simulink model "gm_sampleModel1857_sub"  (R2023a)
settings: Solver=VariableStepAuto  StartTime=0.0  StopTime=10.0  RelTol=1e-3
libraries: simulink x2, hdlsllib x1
settings Model: Creator=user1  LastModifiedBy=user1
settings OptimizationCC: BlockReduction=off  ConditionallyExecuteInputs=off
settings DebuggingCC: InheritedTsInSrcMsg=none

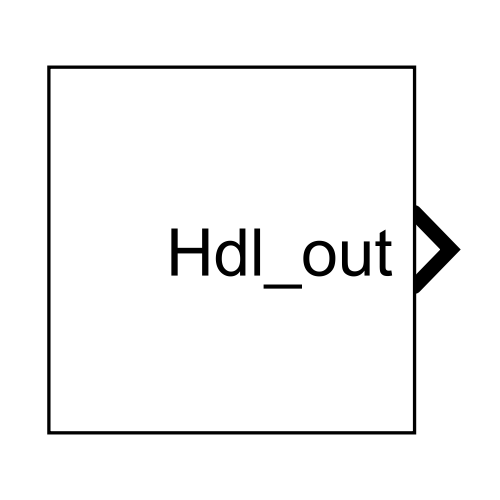
[thumbnail: Simulink's stored preview of the top-level diagram]
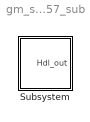
== system gm_sampleModel1857_sub ==
  Subsystem : Subsystem

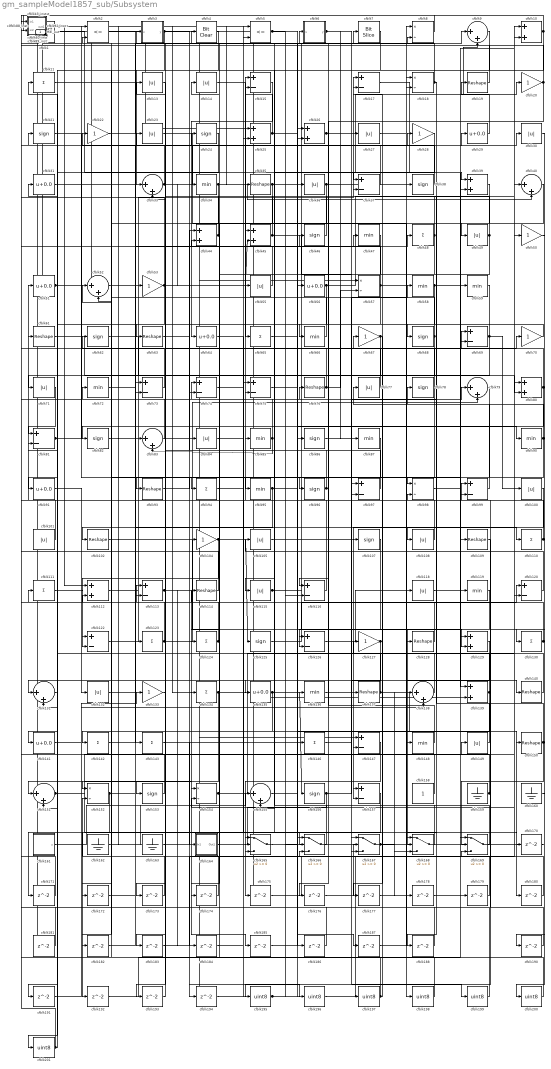
== system gm_sampleModel1857_sub/Subsystem ==
  cfblk1 : simulink/Logic and Bit Operations/Extract Bits  bitsToExtract=Upper half  numBits=8  bitIdxRange=[0 7]  outScalingMode=Preserve fixed-point scaling
      settings: LibrarySourceBlock=|
      | hdlsllib/Logic and Bit
      | Operations/Extract Bits
  cfblk{10,25..26,39,44..45,80,112,129,139} (10 alike) : Sum  OutDataTypeStr=uint8
  cfblk{13..14,23,27,30,36,49,55,71,77,84,100..101,105,108,115,118,132,149} (19 alike) : Abs  OutDataTypeStr=uint8  SaturateOnIntegerOverflow=off
  cfblk{19,35,61,63,76,93,102,109,114,128,137,140,150} (13 alike) : Reshape
  cfblk103_inst : Subsystem
  cfblk{20,22,28,50,53,67,70,104,127,133} (10 alike) : Gain  OutDataTypeStr=uint8
  cfblk{21,24,38,46,62,68,78,82,86,96,107,125,153,156} (14 alike) : Signum
  cfblk{11,48,65,94,110..111,123..124,130,134,142..143,146} (13 alike) : Sum  Inputs=+  OutDataTypeStr=uint8
  cfblk{15,17,37,69,73..75,81,97,99,113,116,120,122,126,147,157} (17 alike) : Sum  Inputs=+-  OutDataTypeStr=uint8
  cfblk117_inst : Subsystem
  cfblk{34,47,58..59,66,72,85,87,90,95,119,136,148} (13 alike) : MinMax  OutDataTypeStr=uint8
  cfblk121_inst : Subsystem
  cfblk12_inst : Subsystem
  cfblk{9,33,40,52,79,83,131,138,151,155} (10 alike) : Sum  Inputs=|++  OutDataTypeStr=uint8
  cfblk{29,31,51,56,64,91,135,141} (8 alike) : Bias  Bias=0.0  SaturateOnIntegerOverflow=off
  cfblk144_inst : Subsystem
  cfblk145_inst : Subsystem
  cfblk{8,18,57,98,152,154} (6 alike) : Product  Inputs=*/  OutDataTypeStr=uint8  RndMeth=Zero  SaturateOnIntegerOverflow=on
  cfblk158 : Constant  OutDataTypeStr=uint8  SampleTime=-1
  cfblk{159..160,162..163} (4 alike) : Ground
  cfblk161 : Subsystem  mask(Counter Limited){uplimit=double(7), tsamp=double(-1)}
      mask prompts: uplimit "Simulink:masks:UpperLimit_MP"; tsamp "Simulink:masks:SampleTime_MP"
      mask help: Simulink:masks:CounterLimited_MD
      mask init:
      | nbits = double(8);
      | tsamp = double(-1);
      | uplimit = double(7);
  cfblk164 : Subsystem
  cfblk{165..169} (5 alike) : Switch  OutDataTypeStr=uint8  SaturateOnIntegerOverflow=off  InputSameDT=off
  cfblk16_inst : Subsystem
  cfblk{170..188,190..194} (24 alike) : Delay  SampleTime=1
  cfblk{195..201} (7 alike) : DataTypeConversion  OutDataTypeStr=uint8  SaturateOnIntegerOverflow=off  RndMeth=Floor
  cfblk2 : RelationalOperator  Operator=<=  OutDataTypeStr=boolean  InputSameDT=off
  cfblk3 : Subsystem  mask(Compare To Zero){relop=<=, OutDataTypeStr=uint8, ZeroCross=on}
      mask prompts: relop "Simulink:masks:Operator_MP"; OutDataTypeStr "Simulink:masks:OutputDataType_MP"; ZeroCross "Simulink:masks:EnableZerocrossingDetection_MP"
      mask help: Simulink:masks:CompareToZero_MD
      mask init:
      | OutDataTypeStr = 'uint8';
      | ZeroCross = 'on';
      | blkName = 'sampleModel1857_sub/Subsystem/cfblk3';
      | relop = '<=';
      | setValue = 'fixdt(0, 8)';
      mask TypeOptions relop: == | ~= | < | <= | >= | >
      mask TypeOptions OutDataTypeStr: Simulink:masks:uint8 | Simulink:masks:boolean
      mask Callback ZeroCross: sl('zeroCrossEnable', gcbh);
      mask Display: disp([relop,' 0'])
  cfblk32_inst : Subsystem
  cfblk4 : simulink/Logic and Bit Operations/Bit Clear  iBit=0
      settings: LibrarySourceBlock=|
      | hdlsllib/Logic and Bit
      | Operations/Bit Clear
  cfblk41_inst : Subsystem
  cfblk42_inst : Subsystem
  cfblk43_inst : Subsystem
  cfblk5 : RelationalOperator  Operator=<=  OutDataTypeStr=boolean  InputSameDT=off
  cfblk6 : Subsystem  mask(Compare To Zero){relop=<=, OutDataTypeStr=uint8, ZeroCross=on}
      mask prompts: relop "Simulink:masks:Operator_MP"; OutDataTypeStr "Simulink:masks:OutputDataType_MP"; ZeroCross "Simulink:masks:EnableZerocrossingDetection_MP"
      mask help: Simulink:masks:CompareToZero_MD
      mask init:
      | OutDataTypeStr = 'uint8';
      | ZeroCross = 'on';
      | blkName = 'sampleModel1857_sub/Subsystem/cfblk6';
      | relop = '<=';
      | setValue = 'fixdt(0, 8)';
      mask TypeOptions relop: == | ~= | < | <= | >= | >
      mask TypeOptions OutDataTypeStr: Simulink:masks:uint8 | Simulink:masks:boolean
      mask Callback ZeroCross: sl('zeroCrossEnable', gcbh);
      mask Display: disp([relop,' 0'])
  cfblk60_inst : Subsystem
  cfblk7 : hdlsllib/Logic and Bit Operations/Bit Slice  lidx=7  ridx=0
  cfblk88_inst : Subsystem
  cfblk89_inst : Subsystem
  cfblk92_inst : Subsystem
  Hdl_out : Outport  OutDataTypeStr=uint8  SampleTime=1
  wires:
  cfblk1/1 -> cfblk39/1
  cfblk10/1 -> cfblk41_inst/2(in2), cfblk33/1
  cfblk100/1 -> cfblk157/2
  cfblk101/1 -> cfblk117_inst/1(in1)
  cfblk102/1 -> cfblk129/2
  cfblk103_inst/1(out1) -> cfblk117_inst/2(in2), cfblk101/1
  cfblk104/1 -> cfblk125/1, cfblk122/2
  cfblk105/1 -> cfblk157/1
  cfblk107/1 -> cfblk126/2
  cfblk108/1 -> cfblk103_inst/1(in1)
  cfblk109/1 -> cfblk195/1
  cfblk11/1 -> cfblk143/1
  cfblk110/1 -> cfblk51/1, cfblk98/2
  cfblk111/1 -> cfblk122/1
  cfblk112/1 -> cfblk48/1
  cfblk113/1 -> cfblk185/1, cfblk184/1
  cfblk114/1 -> cfblk32_inst/1(in1)
  cfblk115/1 -> cfblk7/1, cfblk168/2
  cfblk116/1 -> cfblk15/1
  cfblk117_inst/1(out1) -> cfblk137/1
  cfblk118/1 -> cfblk139/1
  cfblk119/1 -> cfblk166/2
  cfblk12_inst/1(out1) -> cfblk179/1
  cfblk120/1 -> cfblk105/1
  cfblk121_inst/1(out1) -> cfblk164/1(In1)
  cfblk122/1 -> cfblk17/1
  cfblk123/1 -> cfblk79/2, cfblk32_inst/2(in2), cfblk183/1
  cfblk124/1 -> cfblk31/1, cfblk113/1
  cfblk125/1 -> cfblk120/1
  cfblk126/1 -> cfblk118/1
  cfblk127/1 -> cfblk147/2, cfblk131/1
  cfblk128/1 -> cfblk114/1
  cfblk129/1 -> cfblk148/1
  cfblk13/1 -> cfblk93/1
  cfblk130/1 -> cfblk52/2, cfblk128/1
  cfblk131/1 -> cfblk81/2
  cfblk132/1 -> cfblk83/1
  cfblk133/1 -> cfblk23/1
  cfblk134/1 -> cfblk151/2, cfblk18/1
  cfblk135/1 -> cfblk156/1, cfblk116/2, cfblk142/1
  cfblk136/1 -> cfblk140/1
  cfblk137/1 -> cfblk75/2, cfblk168/3, cfblk180/1
  cfblk138/1 -> cfblk6/1(u)
  cfblk139/1 -> cfblk112/2, cfblk173/1
  cfblk14/1 -> cfblk65/1
  cfblk140/1 -> cfblk61/1
  cfblk141/1 -> cfblk133/1
  cfblk142/1 -> cfblk69/1
  cfblk143/1 -> cfblk56/1
  cfblk144_inst/1(out1) -> cfblk147/1
  cfblk145_inst/1(out1) -> cfblk38/1
  cfblk146/1 -> cfblk58/1
  cfblk147/1 -> cfblk175/1
  cfblk148/1 -> cfblk76/1
  cfblk149/1 -> cfblk37/2
  cfblk15/1 -> cfblk64/1
  cfblk150/1 -> cfblk74/1, cfblk169/2
  cfblk151/1 -> cfblk165/3, cfblk120/2, cfblk154/1
  cfblk152/1 -> cfblk73/1, cfblk192/1
  cfblk153/1 -> cfblk72/1
  cfblk154/1 -> cfblk40/1, cfblk59/1
  cfblk155/1 -> cfblk149/1
  cfblk156/1 -> cfblk70/1, cfblk154/2
  cfblk157/1 -> cfblk171/1
  cfblk158/1 -> cfblk111/1
  cfblk159/1 -> cfblk89_inst/2(in2), cfblk16_inst/1(in1)
  cfblk16_inst/1(out1) -> cfblk25/1
  cfblk160/1 -> cfblk200/1
  cfblk161/1(y) -> cfblk5/2
  cfblk162/1 -> cfblk155/1
  cfblk163/1 -> cfblk146/1
  cfblk164/1(Out1) -> cfblk50/1
  cfblk165/1 -> cfblk186/1
  cfblk166/1 -> cfblk41_inst/1(in1)
  cfblk167/1 -> cfblk67/1, cfblk178/1
  cfblk168/1 -> cfblk44/2
  cfblk169/1 -> cfblk85/1
  cfblk17/1 -> cfblk129/1
  cfblk170/1 -> cfblk1/1
  cfblk171/1 -> cfblk145_inst/1(in1)
  cfblk172/1 -> cfblk73/2
  cfblk173/1 -> cfblk52/1
  cfblk174/1 -> cfblk2/2
  cfblk175/1 -> cfblk80/1
  cfblk176/1 -> cfblk167/2
  cfblk177/1 -> cfblk17/2
  cfblk178/1 -> cfblk39/2
  cfblk179/1 -> cfblk166/3
  cfblk18/1 -> cfblk5/1, cfblk168/1
  cfblk180/1 -> cfblk152/2
  cfblk181/1 -> cfblk60_inst/1(in1)
  cfblk182/1 -> cfblk45/1
  cfblk183/1 -> cfblk169/3
  cfblk184/1 -> cfblk25/2
  cfblk185/1 -> cfblk26/2
  cfblk186/1 -> cfblk166/1
  cfblk187/1 -> cfblk18/2
  cfblk188/1 -> cfblk75/1
  cfblk19/1 -> cfblk103_inst/2(in2)
  cfblk190/1 -> cfblk99/1
  cfblk191/1 -> cfblk138/2
  cfblk192/1 -> cfblk169/1
  cfblk193/1 -> cfblk3/1(u)
  cfblk194/1 -> cfblk28/1
  cfblk195/1 -> cfblk86/1, cfblk36/1
  cfblk196/1 -> cfblk109/1
  cfblk197/1 -> cfblk22/1, cfblk127/1
  cfblk198/1 -> cfblk88_inst/1(in1)
  cfblk199/1 -> cfblk88_inst/2(in2)
  cfblk2/1 -> cfblk99/2
  cfblk20/1 -> cfblk96/1, cfblk12_inst/2(in2)
  cfblk200/1 -> cfblk4/1
  cfblk201/1 -> cfblk121_inst/1(in1), cfblk11/1
  cfblk21/1 -> cfblk94/1
  cfblk22/1 -> cfblk8/2
  cfblk23/1 -> cfblk198/1
  cfblk24/1 -> cfblk141/1
  cfblk25/1 -> cfblk150/1, cfblk15/2
  cfblk26/1 -> cfblk9/2, cfblk119/1
  cfblk27/1 -> cfblk8/1
  cfblk28/1 -> cfblk135/1
  cfblk29/1 -> cfblk19/1
  cfblk3/1(y) -> cfblk196/1, cfblk102/1
  cfblk30/1 -> cfblk130/1
  cfblk31/1 -> cfblk123/1
  cfblk32_inst/1(out1) -> cfblk92_inst/2(in2)
  cfblk33/1 -> cfblk92_inst/1(in1), cfblk26/1
  cfblk34/1 -> cfblk74/2, cfblk40/2
  cfblk35/1 -> cfblk115/1, cfblk134/1
  cfblk36/1 -> cfblk113/2, cfblk193/1
  cfblk37/1 -> cfblk42_inst/2(in2)
  cfblk38/1 -> cfblk2/1
  cfblk39/1 -> cfblk49/1
  cfblk4/1 -> cfblk201/1
  cfblk40/1 -> cfblk82/1
  cfblk41_inst/1(out1) -> cfblk53/1
  cfblk42_inst/1(out1) -> cfblk112/1, cfblk181/1
  cfblk43_inst/1(out1) -> cfblk84/1, cfblk139/2
  cfblk44/1 -> cfblk144_inst/1(in1), cfblk12_inst/1(in1)
  cfblk45/1 -> cfblk97/1, cfblk43_inst/1(in1)
  cfblk46/1 -> cfblk35/1
  cfblk47/1 -> cfblk116/1
  cfblk48/1 -> cfblk144_inst/2(in2), cfblk174/1
  cfblk49/1 -> cfblk16_inst/2(in2), cfblk66/1
  cfblk5/1 -> cfblk37/1, cfblk187/1
  cfblk50/1 -> cfblk190/1
  cfblk51/1 -> Hdl_out/1, cfblk95/1
  cfblk52/1 -> cfblk110/1
  cfblk53/1 -> cfblk91/1, cfblk45/2, cfblk121_inst/2(in2), cfblk34/1
  cfblk55/1 -> cfblk89_inst/1(in1)
  cfblk56/1 -> cfblk165/2, cfblk10/2
  cfblk57/1 -> cfblk80/2, cfblk43_inst/2(in2), cfblk131/2
  cfblk58/1 -> cfblk71/1, cfblk10/1
  cfblk59/1 -> cfblk124/1
  cfblk6/1(y) -> cfblk199/1, cfblk87/1
  cfblk60_inst/1(out1) -> cfblk104/1
  cfblk61/1 -> cfblk167/1
  cfblk62/1 -> cfblk138/1
  cfblk63/1 -> cfblk194/1
  cfblk64/1 -> cfblk108/1
  cfblk65/1 -> cfblk9/1
  cfblk66/1 -> cfblk14/1
  cfblk67/1 -> cfblk177/1, cfblk176/1
  cfblk68/1 -> cfblk21/1, cfblk167/3
  cfblk69/1 -> cfblk68/1, cfblk100/1, cfblk191/1
  cfblk7/1 -> cfblk155/2
  cfblk70/1 -> cfblk63/1
  cfblk71/1 -> cfblk81/1
  cfblk72/1 -> cfblk30/1
  cfblk73/1 -> cfblk60_inst/2(in2)
  cfblk74/1 -> cfblk170/1
  cfblk75/1 -> cfblk90/1
  cfblk76/1 -> cfblk55/1, cfblk57/2
  cfblk77/1 -> cfblk46/1
  cfblk78/1 -> cfblk24/1, cfblk153/1
  cfblk79/1 -> cfblk182/1
  cfblk8/1 -> cfblk42_inst/1(in1)
  cfblk80/1 -> cfblk13/1, cfblk172/1
  cfblk81/1 -> cfblk69/2, cfblk27/1
  cfblk82/1 -> cfblk97/2
  cfblk83/1 -> cfblk62/1
  cfblk84/1 -> cfblk29/1
  cfblk85/1 -> cfblk83/2, cfblk145_inst/2(in2)
  cfblk86/1 -> cfblk79/1
  cfblk87/1 -> cfblk165/1
  cfblk88_inst/1(out1) -> cfblk197/1
  cfblk89_inst/1(out1) -> cfblk57/1
  cfblk9/1 -> cfblk151/1
  cfblk90/1 -> cfblk77/1, cfblk188/1
  cfblk91/1 -> cfblk132/1
  cfblk92_inst/1(out1) -> cfblk136/1
  cfblk93/1 -> cfblk98/1
  cfblk94/1 -> cfblk107/1
  cfblk95/1 -> cfblk152/1, cfblk47/1
  cfblk96/1 -> cfblk33/2, cfblk126/1
  cfblk97/1 -> cfblk44/1
  cfblk98/1 -> cfblk20/1
  cfblk99/1 -> cfblk78/1

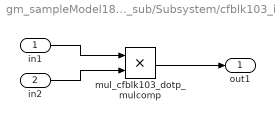
== system gm_sampleModel1857_sub/Subsystem/cfblk103_inst ==
  in1 : Inport  OutDataTypeStr=uint8  SampleTime=1
  in2 : Inport  Port=2  OutDataTypeStr=uint8  SampleTime=1
  mul_cfblk103_dotp_mulcomp : Product  Inputs=**  OutDataTypeStr=uint8  SampleTime=1
  out1 : Outport  OutDataTypeStr=uint8  SampleTime=1
  wires:
  in1/1 -> mul_cfblk103_dotp_mulcomp/1
  in2/1 -> mul_cfblk103_dotp_mulcomp/2
  mul_cfblk103_dotp_mulcomp/1 -> out1/1

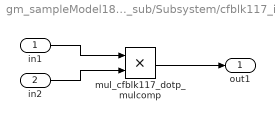
== system gm_sampleModel1857_sub/Subsystem/cfblk117_inst ==
  in1 : Inport  OutDataTypeStr=uint8  SampleTime=1
  in2 : Inport  Port=2  OutDataTypeStr=uint8  SampleTime=1
  mul_cfblk117_dotp_mulcomp : Product  Inputs=**  OutDataTypeStr=uint8  SampleTime=1
  out1 : Outport  OutDataTypeStr=uint8  SampleTime=1
  wires:
  in1/1 -> mul_cfblk117_dotp_mulcomp/1
  in2/1 -> mul_cfblk117_dotp_mulcomp/2
  mul_cfblk117_dotp_mulcomp/1 -> out1/1

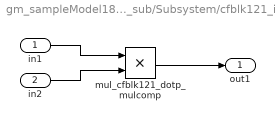
== system gm_sampleModel1857_sub/Subsystem/cfblk121_inst ==
  in1 : Inport  OutDataTypeStr=uint8  SampleTime=1
  in2 : Inport  Port=2  OutDataTypeStr=uint8  SampleTime=1
  mul_cfblk121_dotp_mulcomp : Product  Inputs=**  OutDataTypeStr=uint8  SampleTime=1
  out1 : Outport  OutDataTypeStr=uint8  SampleTime=1
  wires:
  in1/1 -> mul_cfblk121_dotp_mulcomp/1
  in2/1 -> mul_cfblk121_dotp_mulcomp/2
  mul_cfblk121_dotp_mulcomp/1 -> out1/1

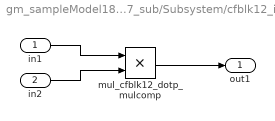
== system gm_sampleModel1857_sub/Subsystem/cfblk12_inst ==
  in1 : Inport  OutDataTypeStr=uint8  SampleTime=1
  in2 : Inport  Port=2  OutDataTypeStr=uint8  SampleTime=1
  mul_cfblk12_dotp_mulcomp : Product  Inputs=**  OutDataTypeStr=uint8  SampleTime=1
  out1 : Outport  OutDataTypeStr=uint8  SampleTime=1
  wires:
  in1/1 -> mul_cfblk12_dotp_mulcomp/1
  in2/1 -> mul_cfblk12_dotp_mulcomp/2
  mul_cfblk12_dotp_mulcomp/1 -> out1/1

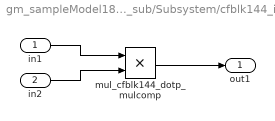
== system gm_sampleModel1857_sub/Subsystem/cfblk144_inst ==
  in1 : Inport  OutDataTypeStr=uint8  SampleTime=1
  in2 : Inport  Port=2  OutDataTypeStr=uint8  SampleTime=1
  mul_cfblk144_dotp_mulcomp : Product  Inputs=**  OutDataTypeStr=uint8  SampleTime=1
  out1 : Outport  OutDataTypeStr=uint8  SampleTime=1
  wires:
  in1/1 -> mul_cfblk144_dotp_mulcomp/1
  in2/1 -> mul_cfblk144_dotp_mulcomp/2
  mul_cfblk144_dotp_mulcomp/1 -> out1/1

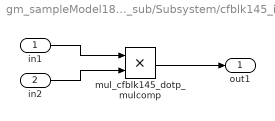
== system gm_sampleModel1857_sub/Subsystem/cfblk145_inst ==
  in1 : Inport  OutDataTypeStr=uint8  SampleTime=1
  in2 : Inport  Port=2  OutDataTypeStr=uint8  SampleTime=1
  mul_cfblk145_dotp_mulcomp : Product  Inputs=**  OutDataTypeStr=uint8  SampleTime=1
  out1 : Outport  OutDataTypeStr=uint8  SampleTime=1
  wires:
  in1/1 -> mul_cfblk145_dotp_mulcomp/1
  in2/1 -> mul_cfblk145_dotp_mulcomp/2
  mul_cfblk145_dotp_mulcomp/1 -> out1/1

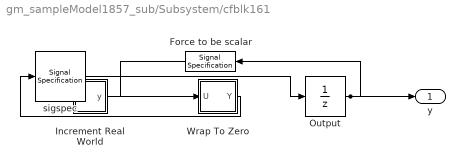
== system gm_sampleModel1857_sub/Subsystem/cfblk161 ==
  Force to be scalar : SignalSpecification  DisableCoverage=on  Dimensions=1
  Increment Real World : Subsystem  mask(Real World Value Increment){}
      mask help: Simulink:masks:RealWorldValueIncrement_MD
      mask Display: disp('V++')
  Output : UnitDelay  InitialCondition=0.0  SampleTime=tsamp  HasFrameUpgradeWarning=on
  Wrap To Zero : Subsystem  mask(Wrap To Zero){Threshold=double(7)}
      mask prompts: Threshold "Simulink:masks:Threshold_MP"
      mask help: Simulink:masks:WrapToZero_MD
  sigspec : SignalSpecification  OutDataTypeStr=uint8  Dimensions=1
  y : Outport  SampleTime=1
  wires:
  Force to be scalar/1 -> Increment Real World/1(u)
  Increment Real World/1(y) -> Wrap To Zero/1(U)
  Output/1 -> Force to be scalar/1, y/1
  Wrap To Zero/1(Y) -> sigspec/1
  sigspec/1 -> Output/1

== system gm_sampleModel1857_sub/Subsystem/cfblk164 ==
  In1 : Inport  OutDataTypeStr=uint8  PortDimensions=1  SampleTime=1
  Out1 : Outport  SampleTime=1
  wires:
  In1/1 -> Out1/1

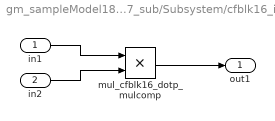
== system gm_sampleModel1857_sub/Subsystem/cfblk16_inst ==
  in1 : Inport  OutDataTypeStr=uint8  SampleTime=1
  in2 : Inport  Port=2  OutDataTypeStr=uint8  SampleTime=1
  mul_cfblk16_dotp_mulcomp : Product  Inputs=**  OutDataTypeStr=uint8  SampleTime=1
  out1 : Outport  OutDataTypeStr=uint8  SampleTime=1
  wires:
  in1/1 -> mul_cfblk16_dotp_mulcomp/1
  in2/1 -> mul_cfblk16_dotp_mulcomp/2
  mul_cfblk16_dotp_mulcomp/1 -> out1/1

== system gm_sampleModel1857_sub/Subsystem/cfblk3 ==
  u : Inport  OutDataTypeStr=uint8  SampleTime=1
  Compare : RelationalOperator  Operator=<=  OutDataTypeStr=fixdt(0, 8)
  Constant : Constant  DisableCoverage=on  Value=0  OutDataTypeStr=Inherit: Inherit via back propagation  SampleTime=-1  PreserveConstantTs=on
  y : Outport  SampleTime=1
  wires:
  u/1 -> Compare/1
  Compare/1 -> y/1
  Constant/1 -> Compare/2

== system gm_sampleModel1857_sub/Subsystem/cfblk32_inst ==
  in1 : Inport  OutDataTypeStr=uint8  SampleTime=1
  in2 : Inport  Port=2  OutDataTypeStr=uint8  SampleTime=1
  mul_cfblk32_dotp_mulcomp : Product  Inputs=**  OutDataTypeStr=uint8  SampleTime=1
  out1 : Outport  OutDataTypeStr=uint8  SampleTime=1
  wires:
  in1/1 -> mul_cfblk32_dotp_mulcomp/1
  in2/1 -> mul_cfblk32_dotp_mulcomp/2
  mul_cfblk32_dotp_mulcomp/1 -> out1/1

== system gm_sampleModel1857_sub/Subsystem/cfblk41_inst ==
  in1 : Inport  OutDataTypeStr=uint8  SampleTime=1
  in2 : Inport  Port=2  OutDataTypeStr=uint8  SampleTime=1
  mul_cfblk41_dotp_mulcomp : Product  Inputs=**  OutDataTypeStr=uint8  SampleTime=1
  out1 : Outport  OutDataTypeStr=uint8  SampleTime=1
  wires:
  in1/1 -> mul_cfblk41_dotp_mulcomp/1
  in2/1 -> mul_cfblk41_dotp_mulcomp/2
  mul_cfblk41_dotp_mulcomp/1 -> out1/1

== system gm_sampleModel1857_sub/Subsystem/cfblk42_inst ==
  in1 : Inport  OutDataTypeStr=uint8  SampleTime=1
  in2 : Inport  Port=2  OutDataTypeStr=uint8  SampleTime=1
  mul_cfblk42_dotp_mulcomp : Product  Inputs=**  OutDataTypeStr=uint8  SampleTime=1
  out1 : Outport  OutDataTypeStr=uint8  SampleTime=1
  wires:
  in1/1 -> mul_cfblk42_dotp_mulcomp/1
  in2/1 -> mul_cfblk42_dotp_mulcomp/2
  mul_cfblk42_dotp_mulcomp/1 -> out1/1

== system gm_sampleModel1857_sub/Subsystem/cfblk43_inst ==
  in1 : Inport  OutDataTypeStr=uint8  SampleTime=1
  in2 : Inport  Port=2  OutDataTypeStr=uint8  SampleTime=1
  mul_cfblk43_dotp_mulcomp : Product  Inputs=**  OutDataTypeStr=uint8  SampleTime=1
  out1 : Outport  OutDataTypeStr=uint8  SampleTime=1
  wires:
  in1/1 -> mul_cfblk43_dotp_mulcomp/1
  in2/1 -> mul_cfblk43_dotp_mulcomp/2
  mul_cfblk43_dotp_mulcomp/1 -> out1/1

== system gm_sampleModel1857_sub/Subsystem/cfblk6 ==
  u : Inport  OutDataTypeStr=uint8  SampleTime=1
  Compare : RelationalOperator  Operator=<=  OutDataTypeStr=fixdt(0, 8)
  Constant : Constant  DisableCoverage=on  Value=0  OutDataTypeStr=Inherit: Inherit via back propagation  SampleTime=-1  PreserveConstantTs=on
  y : Outport  SampleTime=1
  wires:
  u/1 -> Compare/1
  Compare/1 -> y/1
  Constant/1 -> Compare/2

== system gm_sampleModel1857_sub/Subsystem/cfblk60_inst ==
  in1 : Inport  OutDataTypeStr=uint8  SampleTime=1
  in2 : Inport  Port=2  OutDataTypeStr=uint8  SampleTime=1
  mul_cfblk60_dotp_mulcomp : Product  Inputs=**  OutDataTypeStr=uint8  SampleTime=1
  out1 : Outport  OutDataTypeStr=uint8  SampleTime=1
  wires:
  in1/1 -> mul_cfblk60_dotp_mulcomp/1
  in2/1 -> mul_cfblk60_dotp_mulcomp/2
  mul_cfblk60_dotp_mulcomp/1 -> out1/1

== system gm_sampleModel1857_sub/Subsystem/cfblk88_inst ==
  in1 : Inport  OutDataTypeStr=uint8  SampleTime=1
  in2 : Inport  Port=2  OutDataTypeStr=uint8  SampleTime=1
  mul_cfblk88_dotp_mulcomp : Product  Inputs=**  OutDataTypeStr=uint8  SampleTime=1
  out1 : Outport  OutDataTypeStr=uint8  SampleTime=1
  wires:
  in1/1 -> mul_cfblk88_dotp_mulcomp/1
  in2/1 -> mul_cfblk88_dotp_mulcomp/2
  mul_cfblk88_dotp_mulcomp/1 -> out1/1

== system gm_sampleModel1857_sub/Subsystem/cfblk89_inst ==
  in1 : Inport  OutDataTypeStr=uint8  SampleTime=1
  in2 : Inport  Port=2  OutDataTypeStr=uint8  SampleTime=1
  mul_cfblk89_dotp_mulcomp : Product  Inputs=**  OutDataTypeStr=uint8  SampleTime=1
  out1 : Outport  OutDataTypeStr=uint8  SampleTime=1
  wires:
  in1/1 -> mul_cfblk89_dotp_mulcomp/1
  in2/1 -> mul_cfblk89_dotp_mulcomp/2
  mul_cfblk89_dotp_mulcomp/1 -> out1/1

== system gm_sampleModel1857_sub/Subsystem/cfblk92_inst ==
  in1 : Inport  OutDataTypeStr=uint8  SampleTime=1
  in2 : Inport  Port=2  OutDataTypeStr=uint8  SampleTime=1
  mul_cfblk92_dotp_mulcomp : Product  Inputs=**  OutDataTypeStr=uint8  SampleTime=1
  out1 : Outport  OutDataTypeStr=uint8  SampleTime=1
  wires:
  in1/1 -> mul_cfblk92_dotp_mulcomp/1
  in2/1 -> mul_cfblk92_dotp_mulcomp/2
  mul_cfblk92_dotp_mulcomp/1 -> out1/1

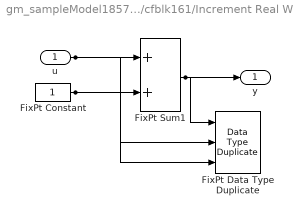
== system gm_sampleModel1857_sub/Subsystem/cfblk161/Increment Real World ==
  u : Inport  OutDataTypeStr=uint8  SampleTime=1
  FixPt Constant : Constant  DisableCoverage=on  OutDataTypeStr=Inherit: Inherit via back propagation  SampleTime=-1
  FixPt Data Type Duplicate : DataTypeDuplicate  DisableCoverage=on  NumInputPorts=3
  FixPt Sum1 : Sum  InputSameDT=on  OutDataTypeStr=Inherit: Inherit via back propagation  LockScale=on
  y : Outport  SampleTime=1
  wires:
  u/1 -> FixPt Sum1/1, FixPt Data Type Duplicate/2
  FixPt Constant/1 -> FixPt Sum1/2, FixPt Data Type Duplicate/3
  FixPt Sum1/1 -> FixPt Data Type Duplicate/1, y/1

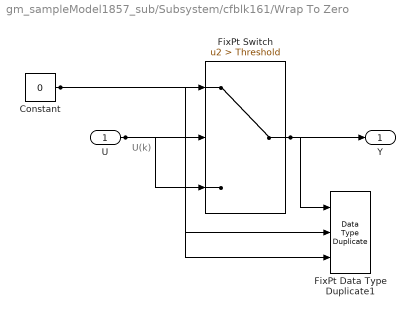
== system gm_sampleModel1857_sub/Subsystem/cfblk161/Wrap To Zero ==
  note: U(k)
  U : Inport  OutDataTypeStr=uint8  SampleTime=1
  Constant : Constant  DisableCoverage=on  Value=0  OutDataTypeStr=Inherit: Inherit via back propagation  SampleTime=-1
  FixPt Data Type Duplicate1 : DataTypeDuplicate  DisableCoverage=on  NumInputPorts=3
  FixPt Switch : Switch  Criteria=u2 > Threshold  Threshold=Threshold  OutDataTypeStr=Inherit: Inherit via back propagation  ZeroCross=off  SaturateOnIntegerOverflow=off  InputSameDT=off
  Y : Outport  SampleTime=1
  wires:
  U/1 -> FixPt Switch/3, FixPt Switch/2, FixPt Data Type Duplicate1/2
  Constant/1 -> FixPt Switch/1, FixPt Data Type Duplicate1/3
  FixPt Switch/1 -> FixPt Data Type Duplicate1/1, Y/1
